simulink model "state_fb_model_v5"  (R2019a)
settings: Solver=ode4  StartTime=0.0  StopTime=endtime  FixedStep=0.001  RelTol=1e-3
undefined symbols (not defined in the file or in its folder): Bd, K
settings Model: Creator=chris  LastModifiedBy=chris

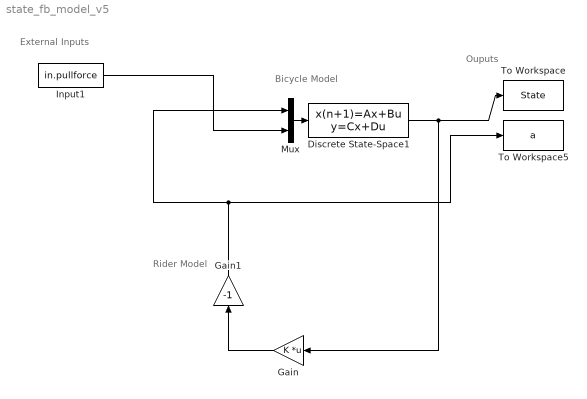
== system state_fb_model_v5 ==
  note: Bicycle Model
  note: External Inputs
  note: Rider Model
  note: Ouputs
  Discrete State-Space1 : DiscreteStateSpace  A=Bd.A  B=Bd.B  C=Bd.C  D=Bd.D  SampleTime=-1
  Gain : Gain  Gain=K  Multiplication=Matrix(K*u) (u vector)
  Gain1 : Gain  Gain=-1
  Input1 : FromWorkspace  VariableName=in.pullforce  SampleTime=0
  Mux : Mux  Inputs=2
  To Workspace : ToWorkspace  VariableName=State  SampleTime=-1
  To Workspace5 : ToWorkspace  VariableName=a  SampleTime=-1
  wires:
  Gain1/1 -> Mux/1, To Workspace5/1
  Mux/1 -> Discrete State-Space1/1
  Input1/1 -> Mux/2
  Gain/1 -> Gain1/1
  Discrete State-Space1/1 -> Gain/1, To Workspace/1
